simulink model "AFS_curvature_reference_backup"  (R2025b)
settings: Solver=VariableStepAuto  StartTime=0.0  StopTime=10.0  RelTol=1e-3
undefined symbols (not defined in the file): afs, dspblkCoreblockFVToolHelper, gcbh, solveAFSMPCOnline
settings Model: Creator=jaiden  LastModifiedBy=r3anjum

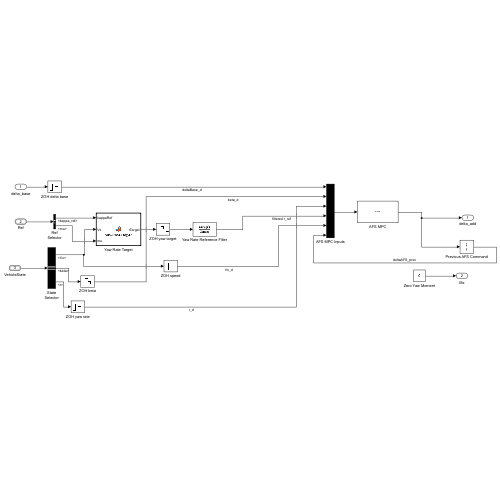
[thumbnail: Simulink's stored preview of the top-level diagram]
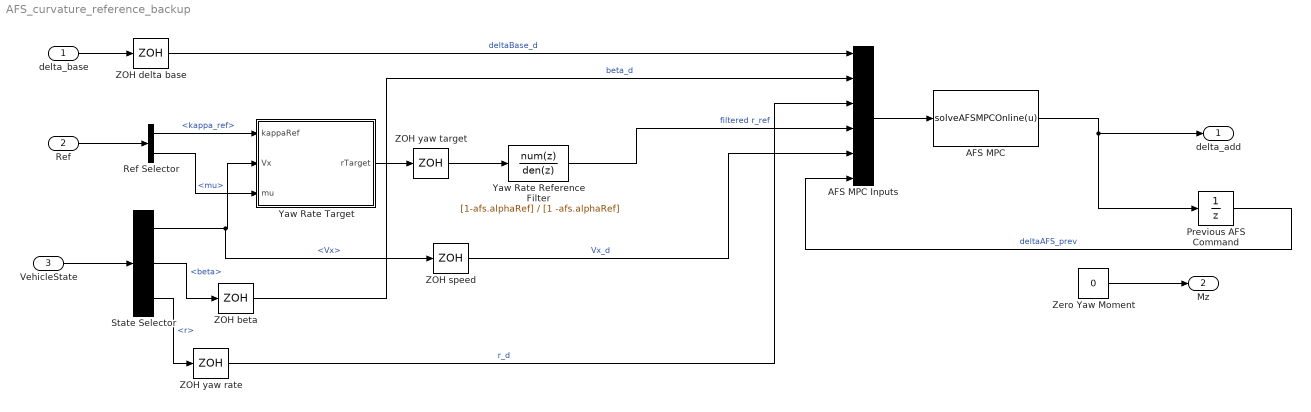
== system AFS_curvature_reference_backup ==
  delta_base : Inport
  Ref : Inport  Port=2  OutDataTypeStr=Bus: ReferenceBus
  VehicleState : Inport  Port=3  OutDataTypeStr=Bus: VehicleStateBus
  AFS MPC : MATLABFcn  MATLABFcn=solveAFSMPCOnline(u)  OutputDimensions=1  OutputSignalType=real
  AFS MPC Inputs : Mux  Inputs=6
  Previous AFS Command : UnitDelay  SampleTime=afs.Ts  HasFrameUpgradeWarning=on
  Ref Selector : BusSelector  OutputSignals=kappa_ref,mu
  State Selector : BusSelector  OutputSignals=Vx,beta,r
  Yaw Rate Reference Filter : DiscreteTransferFcn  LoadFcn=dspblkCoreblockFVToolHelper(gcbh,'load');  Numerator=[1-afs.alphaRef]  Denominator=[1 -afs.alphaRef]
      settings: CopyFcn=dspblkCoreblockFVToolHelper(gcbh,'copy');  DeleteFcn=dspblkCoreblockFVToolHelper(gcbh,'close');  ModelCloseFcn=dspblkCoreblockFVToolHelper(gcbh,'close');  PreSaveFcn=dspblkCoreblockFVToolHelper(gcbh,'presave');  PostSaveFcn=dspblkCoreblockFVToolHelper(gcbh,'postsave');  CloseFcn=dspblkCoreblockFVToolHelper(gcbh,'close');
  Yaw Rate Target : MATLAB Function  TreatAsAtomicUnit=on
  ZOH beta : ZeroOrderHold  SampleTime=afs.Ts
  ZOH delta base : ZeroOrderHold  SampleTime=afs.Ts
  ZOH speed : ZeroOrderHold  SampleTime=afs.Ts
  ZOH yaw rate : ZeroOrderHold  SampleTime=afs.Ts
  ZOH yaw target : ZeroOrderHold  SampleTime=afs.Ts
  Zero Yaw Moment : Constant  Value=0
  delta_add : Outport
  Mz : Outport  Port=2
  wires:
  Ref/1 -> Ref Selector/1
  VehicleState/1 -> State Selector/1
  Ref Selector/1 -> Yaw Rate Target/1(kappaRef)  "<kappa_ref>"
  State Selector/1 -> ZOH speed/1, Yaw Rate Target/2(Vx)  "<Vx>"
  Ref Selector/2 -> Yaw Rate Target/3(mu)  "<mu>"
  Yaw Rate Target/1(rTarget) -> ZOH yaw target/1
  ZOH yaw target/1 -> Yaw Rate Reference Filter/1
  delta_base/1 -> ZOH delta base/1
  State Selector/2 -> ZOH beta/1  "<beta>"
  State Selector/3 -> ZOH yaw rate/1  "<r>"
  ZOH delta base/1 -> AFS MPC Inputs/1  "deltaBase_d"
  ZOH beta/1 -> AFS MPC Inputs/2  "beta_d"
  ZOH yaw rate/1 -> AFS MPC Inputs/3  "r_d"
  Yaw Rate Reference Filter/1 -> AFS MPC Inputs/4  "filtered r_ref"
  ZOH speed/1 -> AFS MPC Inputs/5  "Vx_d"
  Previous AFS Command/1 -> AFS MPC Inputs/6  "deltaAFS_prev"
  AFS MPC Inputs/1 -> AFS MPC/1
  Zero Yaw Moment/1 -> Mz/1
  AFS MPC/1 -> Previous AFS Command/1, delta_add/1

== matlab function AFS_curvature_reference_backup/Yaw Rate Target ==
  data: kappaRef input; rTarget output; Vx input; mu input
function rTarget = yawRateTarget(kappaRef, Vx, mu)
%#codegen

g = 9.81;

Vsafe = max(abs(Vx), 0.1);

% Yaw rate required by the road curvature.
rPath = Vx*kappaRef;

% Approximate tire-friction yaw-rate limit.
rLimit = max(mu, 0)*g/Vsafe;

rTarget = min(max(rPath, -rLimit), rLimit);

end
